simulink model "Pruefungsaufgabe_10"  (R2017b)
settings: Solver=ode45  StartTime=0  StopTime=50  MaxStep=1e-3  RelTol=1e-3  EnableMultiTasking=on
values from neighbouring files (symbols this model uses):
  CM = 7.1E-7    (= 7.1e-07)    [Pruefungsaufgabe_10_Konstanten.m]
  Jges = JR + JL    (= 0.00100132)    [Pruefungsaufgabe_10_Konstanten.m]    (also in Pruefungsaufgabe_13_Konstanten.m = 1e-07)
  KM = 38.4E-3    (= 0.0384)    [Pruefungsaufgabe_10_Konstanten.m]    (also in Pruefungsaufgabe_13_Konstanten.m = 0.05; Pruefungsaufgabe_15_Konstanten.m = 0.05)
  KN = 1.5    [Pruefungsaufgabe_10_Konstanten.m]
  LA = 4.64E-4    (= 0.000464)    [Pruefungsaufgabe_10_Konstanten.m]    (also in Pruefungsaufgabe_13_Konstanten.m = 0.0002)
  RA = 4.99    [Pruefungsaufgabe_10_Konstanten.m]    (also in Pruefungsaufgabe_13_Konstanten.m = 0.6; Pruefungsaufgabe_15_Konstanten.m = 5)
libraries: simulink x1
settings Model: Creator=jbaur  LastModifiedBy=jbaur
settings DataIOCC: ExternalInput=X1  SaveFormat=StructureWithTime  InspectSignalLogs=on  SignalLoggingName=sigsOut
settings OptimizationCC: ExpressionDepthLimit=2147483647  InitFltsAndDblsToZero=on  LifeSpan=inf
settings DebuggingCC: SaveWithParameterizedLinksMsg=none  SignalResolutionControl=TryResolveAllWithWarning  MultiTaskDSMMsg=warning  MultiTaskCondExecSysMsg=none  StateNameClashWarn=warning  SFUnexpectedBacktrackingDiag=warning  SFNoUnconditionalDefaultTransitionDiag=warning  SFExecutionAtInitializationDiag=none
settings HardwareCC: ProdBitPerPointer=32  ProdBitPerSizeT=32  ProdBitPerPtrDiffT=32  ProdLargestAtomicFloat=None  ProdIntDivRoundTo=Undefined  ProdEndianess=Unspecified  ProdWordSize=32  ProdHWDeviceType=32-bit Generic  TargetUnknown=on
settings ModelReferenceCC: PropagateSignalLabelsOutOfModel=off
settings CodeAppCC: StateflowObjectComments=on
settings GRTTargetCC: TargetFcnLib=ansi_tfl_tmw.mat  TargetLangStandard=C89/C90 (ANSI)  ModelReferenceCompliant=off  GeneratePreprocessorConditionals=Disable all  CombineOutputUpdateFcns=off  MatFileLogging=off  GRTInterface=on
settings ConfigComp: CovMetricSettings=dw  CovHtmlReporting=on  CovSaveCumulativeToWorkspaceVar=on  CovSaveSingleToWorkspaceVar=on  CovExternalEMLEnable=off  CovSFcnEnable=off

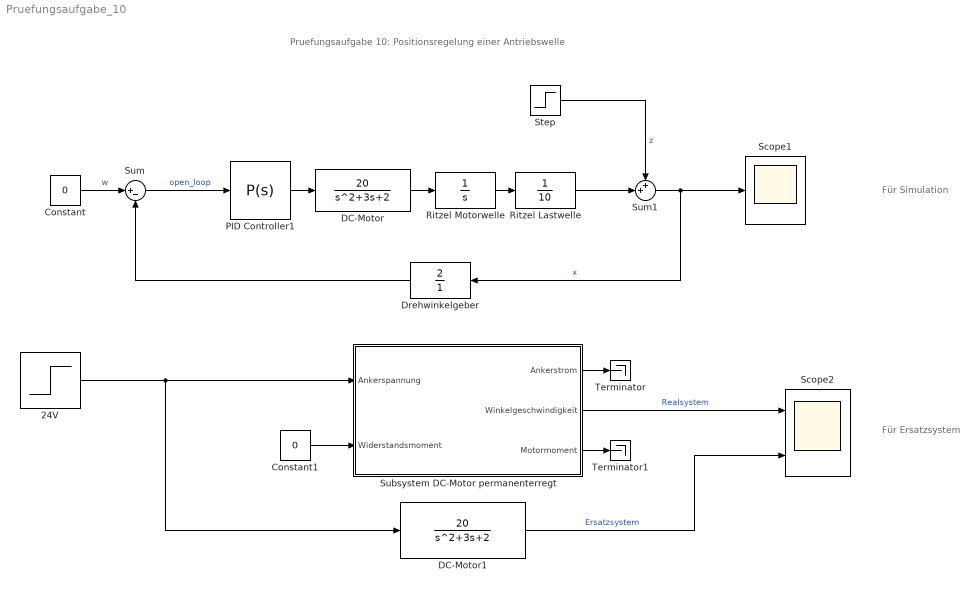
== system Pruefungsaufgabe_10 ==
  note: Pruefungsaufgabe 10: Positionsregelung einer Antriebswelle
  note: Für Simulation
  note: Für Ersatzsystem
  24V : Step  Time=0  After=24  SampleTime=0
  Constant : Constant  Value=0
  Constant1 : Constant  Value=0
  DC-Motor : TransferFcn  Numerator=[20]  Denominator=[1 3 2]
  DC-Motor1 : TransferFcn  Numerator=[20]  Denominator=[1 3 2]
  Drehwinkelgeber : TransferFcn  Numerator=[2]  Denominator=[1]
  PID Controller1 : simulink/Continuous/PID Controller  Controller=P  TimeDomain=Continuous-time  SampleTime=-1  IntegratorMethod=Forward Euler  FilterMethod=Forward Euler  Form=Ideal  UseFilter=on  ControllerParametersSource=internal  P=0.4  I=1  D=0  N=100  InitialConditionSource=internal  InitialConditionForIntegrator=0  InitialConditionForFilter=0  ExternalReset=none  LimitOutput=off  UpperSaturationLimit=inf  LowerSaturationLimit=-inf  LinearizeAsGain=on  AntiWindupMode=none  Kb=1  TrackingMode=off  Kt=1  PParamMin=[]  PParamMax=[]  IParamMin=[]  IParamMax=[]  DParamMin=[]  DParamMax=[]  NParamMin=[]  NParamMax=[]  KbParamMin=[]  KbParamMax=[]  KtParamMin=[]  KtParamMax=[]  POutMin=[]  POutMax=[]  IOutMin=[]  IOutMax=[]  DOutMin=[]  DOutMax=[]  NOutMin=[]  NOutMax=[]  KbOutMin=[]  KbOutMax=[]  KtOutMin=[]  KtOutMax=[]  IntegratorOutMin=[]  IntegratorOutMax=[]  FilterOutMin=[]  FilterOutMax=[]  SumOutMin=[]  SumOutMax=[]  SumI1OutMin=[]  SumI1OutMax=[]  SumI2OutMin=[]  SumI2OutMax=[]  SumI3OutMin=[]  SumI3OutMax=[]  SumDOutMin=[]  SumDOutMax=[]  SaturationOutMin=[]  SaturationOutMax=[]  IntegratorContinuousStateAttributes=''  IntegratorStateMustResolveToSignalObject=off  IntegratorRTWStateStorageClass=Auto  FilterContinuousStateAttributes=''  FilterStateMustResolveToSignalObject=off  FilterRTWStateStorageClass=Auto  DifferentiatorICPrevScaledInput=0  DifferentiatorOutMin=[]  DifferentiatorOutMax=[]  InitialConditionSetting=State (most efficient)  FilterDiffOutCoefMin=[]  FilterDiffOutCoefMax=[]  SumDenOutMin=[]  SumDenOutMax=[]  SumNumOutMin=[]  SumNumOutMax=[]  ReciprocalOutMin=[]  ReciprocalOutMax=[]  DivideOutMin=[]  DivideOutMax=[]  TunerSelectOption=Transfer Function Based (PID Tuner App)
  Ritzel Lastwelle : TransferFcn  Denominator=[10]
  Ritzel Motorwelle : TransferFcn  Denominator=[1 0]
  Scope1 : Scope
  Scope2 : Scope  NumInputPorts=2
  Step : Step  Time=0  SampleTime=0
  Subsystem DC-Motor permanenterregt : Subsystem
  Sum : Sum  Inputs=|+-
  Sum1 : Sum  Inputs=++|
  Terminator : Terminator
  Terminator1 : Terminator
  wires:
  Sum/1 -> PID Controller1/1  "open_loop"
  PID Controller1/1 -> DC-Motor/1
  Constant/1 -> Sum/1  "w"
  DC-Motor/1 -> Ritzel Motorwelle/1
  24V/1 -> Subsystem DC-Motor permanenterregt/1(Ankerspannung), DC-Motor1/1
  Subsystem DC-Motor permanenterregt/2(Winkelgeschwindigkeit) -> Scope2/1  "Realsystem"
  DC-Motor1/1 -> Scope2/2  "Ersatzsystem"
  Ritzel Motorwelle/1 -> Ritzel Lastwelle/1
  Ritzel Lastwelle/1 -> Sum1/2
  Sum1/1 -> Scope1/1, Drehwinkelgeber/1  "x"
  Step/1 -> Sum1/1  "z"
  Drehwinkelgeber/1 -> Sum/2
  Subsystem DC-Motor permanenterregt/1(Ankerstrom) -> Terminator/1
  Subsystem DC-Motor permanenterregt/3(Motormoment) -> Terminator1/1
  Constant1/1 -> Subsystem DC-Motor permanenterregt/2(Widerstandsmoment)

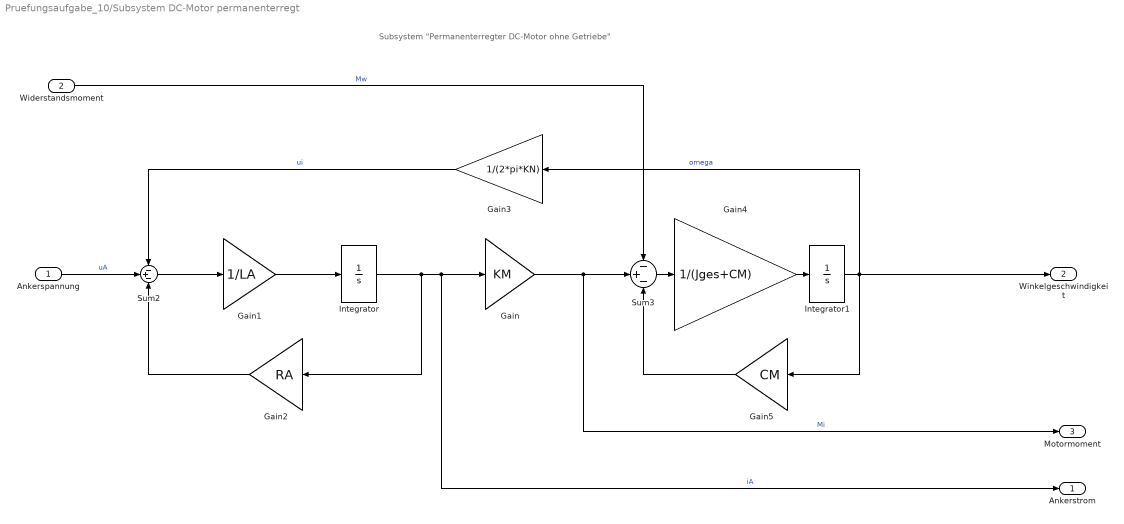
== system Pruefungsaufgabe_10/Subsystem DC-Motor permanenterregt ==
  note: Subsystem "Permanenterregter DC-Motor ohne Getriebe"
  Ankerspannung : Inport
  Widerstandsmoment : Inport  Port=2
  Gain : Gain  Gain=KM
  Gain1 : Gain  Gain=1/LA
  Gain2 : Gain  Gain=RA
  Gain3 : Gain  Gain=1/(2*pi*KN)
  Gain4 : Gain  Gain=1/(Jges+CM)
  Gain5 : Gain  Gain=CM
  Integrator : Integrator
  Integrator1 : Integrator
  Sum2 : Sum  Inputs=-+-
  Sum3 : Sum  Inputs=-+-
  Ankerstrom : Outport
  Winkelgeschwindigkeit : Outport  Port=2
  Motormoment : Outport  Port=3
  wires:
  Ankerspannung/1 -> Sum2/2  "uA"
  Gain3/1 -> Sum2/1  "ui"
  Gain/1 -> Sum3/2, Motormoment/1  "Mi"
  Sum2/1 -> Gain1/1
  Gain1/1 -> Integrator/1
  Integrator/1 -> Gain2/1, Ankerstrom/1, Gain/1  "iA"
  Sum3/1 -> Gain4/1
  Gain4/1 -> Integrator1/1
  Integrator1/1 -> Winkelgeschwindigkeit/1, Gain3/1, Gain5/1  "omega"
  Gain5/1 -> Sum3/3
  Gain2/1 -> Sum2/3
  Widerstandsmoment/1 -> Sum3/1  "Mw"
